simulink model "DCMotor"  (R2019a)
settings: Solver=ode45  StartTime=0.0  StopTime=2  RelTol=1e-3
undefined symbols (not defined in the file): sigbuilder_block
settings Model: Creator=raca  LastModifiedBy=headl
settings DataIOCC: ReturnWorkspaceOutputs=off
settings DebuggingCC: ArithmeticOperatorsInVariantConditions=warning
settings SFSimCC: SimUseLocalCustomCode=off
settings RTWCC: RTWUseLocalCustomCode=off
settings CodeAppCC: StateflowObjectComments=on

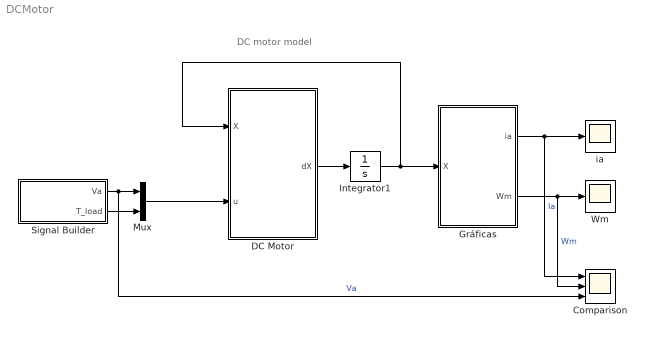
== system DCMotor ==
  note: DC motor model
  Comparison : Scope  NumInputPorts=3
  DC Motor : MATLAB Function  TreatAsAtomicUnit=on
  Gráficas : MATLAB Function  TreatAsAtomicUnit=on
  Integrator1 : Integrator  InitialCondition=[0 0.1]
  Mux : Mux  Inputs=2
  Signal Builder : Subsystem  Tag=STV Subsys  LoadFcn=sigbuilder_block('load');  StartFcn=sigbuilder_block('start');  StopFcn=sigbuilder_block('stop');  ClipboardFcn=sigbuilder_block('clipboard');  mask(Sigbuilder block){tuvar=[0:10]}
      mask help: Simulink:masks:SigbuilderBlock_MD
      mask init:
      | if ~strcmp(get_param(bdroot(gcbh),'SimulationStatus'),'stopped') tuvar = sigbuilder_block('maskInit'); end
      settings: CopyFcn=sigbuilder_block('copy');  DeleteFcn=sigbuilder_block('delete');  ModelCloseFcn=sigbuilder_block('modelClose');  PreSaveFcn=sigbuilder_block('preSave');  PauseFcn=sigbuilder_block('pause');  ContinueFcn=sigbuilder_block('continue');  NameChangeFcn=sigbuilder_block('namechange');  OpenFcn=sigbuilder_block('open',[352.8 97.2 550.8 400.2 ]);  CloseFcn=sigbuilder_block('close');
      mask Display: plot(0, 0, 100, 100,[2, 2, 32, 32, 2], [68, 8, 8, 68, 68],[32, 2], [38, 38], [32, 19, 2],[53, 60, 44], [32, 17, 17, 2],[16, 16, 31, 31]);txt = getActiveGroup(gcbh);text(2, 100, txt,'verticalAlignment', 'top');
  Wm : Scope
  ia : Scope
  wires:
  DC Motor/1(dX) -> Integrator1/1
  Integrator1/1 -> DC Motor/1(X), Gráficas/1(X)
  Gráficas/1(ia) -> Comparison/1, ia/1  "Ia"
  Gráficas/2(Wm) -> Comparison/2, Wm/1  "Wm"
  Mux/1 -> DC Motor/2(u)
  Signal Builder/2(T_load) -> Mux/2
  Signal Builder/1(Va) -> Comparison/3, Mux/1  "Va"

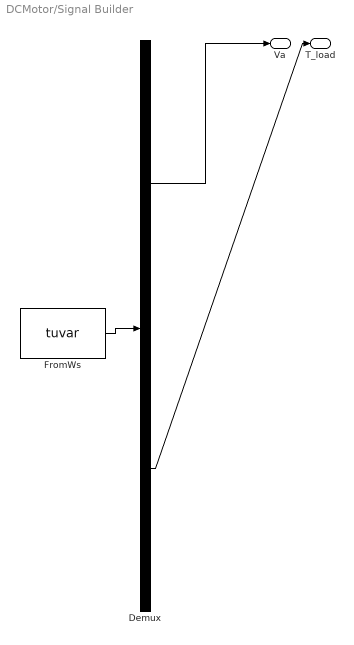
== system DCMotor/Signal Builder ==
  Demux : Demux  Tag=STV Demux  Outputs=2
  FromWs : FromWorkspace  Tag=STV FromWs  VariableName=tuvar  SampleTime=0
      SigBuilderData=|
      | common.afterFinalStr = 'Extrapolate'
      | common.sampleTime = 0
      | dataSet.timeRange = [0 10]
      | dataSet.name = 'Group 1'
      | sbobj.Groups.Name = 'Group 1'
      | sbobj.Groups.Signals(1).Name = 'Va'
      | sbobj.Groups.Signals(1).XData = [0 10]
      | sbobj.Groups.Signals(1).YData = [420 420]
      | sbobj.Groups.Signals(2).Name = 'T_load'
      | sbobj.Groups.Signals(2).XData = [0 10]
      | sbobj.Groups.Signals(2).YData = [430 430]
  Va : Outport  Tag=STV Outport
  T_load : Outport  Tag=STV Outport  Port=2
  wires:
  Demux/1 -> Va/1
  FromWs/1 -> Demux/1
  Demux/2 -> T_load/1

== matlab function DCMotor/DC Motor ==
  data: X input; dX output; u input
% L.Arturo Torres-Romero

function dX = fcn(X,u)
ia = X(1); wm= X(2);
Va = u(1); Tl = u(2);

Ra = 0.193;      % is the equivalent resistance.
La = 3.83e-3;    % is the inductance of the coil.
Jm = 0.6;        % kg/m^2 is the moment of inertia or rotational inertia
bm = 2.632177;   % damping torque coefficient.
Kb = 2.332232;   % anular velocity-Back EMF coefficent.
KT = 2.1717;     % current-torque coefficient.

A = [-Ra/La -Kb/La;KT/Jm -bm/Jm];
B = [1/La 0;0 -1/Jm];


a = A*X;
b = B*u;
dX = A*X + B*u;

end

== matlab function DCMotor/Gráficas ==
  data: X input; ia output; Wm output
function [ia,Wm] = DEMUX(X)
ia = X(1); Wm = X(2);
